simulink model "LQR_Metodo_Simulink"  (R2022a)
settings: Solver=VariableStepAuto  StartTime=0.0  StopTime=2  RelTol=1e-3
undefined symbols (not defined in the file): A, B, C, K, Ke, Kf, Kf_t
settings Model: Creator=gabri  LastModifiedBy=gabri

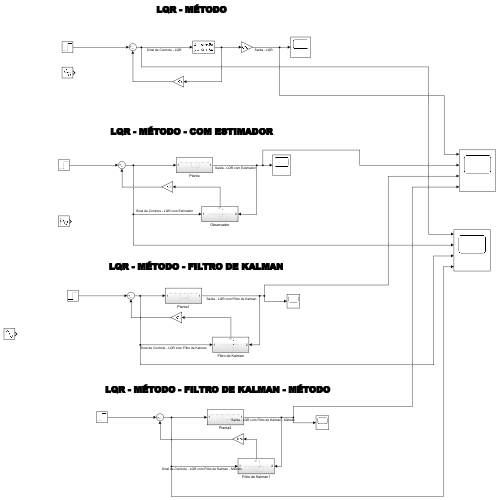
[thumbnail: Simulink's stored preview of the top-level diagram]
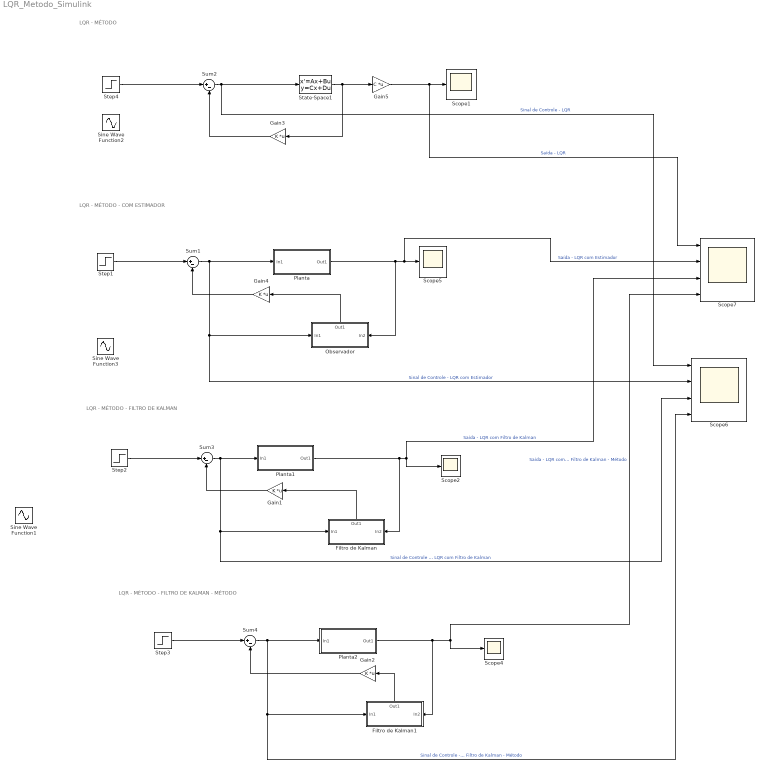
== system LQR_Metodo_Simulink ==
  note: LQR - MÉTODO
  note: LQR - MÉTODO - COM ESTIMADOR
  note: LQR - MÉTODO - FILTRO DE KALMAN
  note: LQR - MÉTODO - FILTRO DE KALMAN - MÉTODO
  Filtro de Kalman : Subsystem
      settings: PortSchema="{\"entries\":[{\"content\":{\"sides\":[{\"content\":{\"connectorIds\":[\"In1\"]},\"type\":\"ConnectorPlacement.EquallySpacedRectSide\",\"uuid\":\"a39a08db-6117-4f96-90c3-02f1f7ffb9ec\"},{\"content\":{\"connectorIds\":[\"In2\"],\"side\":\"RIGHT\"},\"type\":\"ConnectorPlacement.EquallySpacedRectSide\",\"uuid\":\"e0a0a54b-1f6f-4425-9f49-01d22204810c\"},{\"content\":{\"connectorIds\":[\"Out1\"],\"side\":\"TOP\"},\"type\":\"ConnectorPlacement.EquallySpacedRectSide\",\"uuid\":\"f9c2d93e-7541-4a9e-b077-600f0b58f20b\"},{\"content\":{\"connectorIds\":[],\"side\":\"BOTTOM\"},\"type\":\"ConnectorPlacement.EquallySpacedRectSide\",\"uuid\":\"2e0212ac-38a2-465c-9330-e4bad70b5dfc\"}]},\"type\":\"ConnectorPlacement.EquallySpacedConnector\",\"uuid\":\"106c2d4c-b59c-4d15-84b9-899fdea4a460\"}],\"packageUris\":[\"http://schema.mathworks.com/mf0/Connector/R2020b\"],\"version\":\"1.0\"}"
  Filtro de Kalman1 : Subsystem
      settings: PortSchema="{\"entries\":[{\"content\":{\"sides\":[{\"content\":{\"connectorIds\":[\"In1\"]},\"type\":\"ConnectorPlacement.EquallySpacedRectSide\",\"uuid\":\"a39a08db-6117-4f96-90c3-02f1f7ffb9ec\"},{\"content\":{\"connectorIds\":[\"In2\"],\"side\":\"RIGHT\"},\"type\":\"ConnectorPlacement.EquallySpacedRectSide\",\"uuid\":\"e0a0a54b-1f6f-4425-9f49-01d22204810c\"},{\"content\":{\"connectorIds\":[\"Out1\"],\"side\":\"TOP\"},\"type\":\"ConnectorPlacement.EquallySpacedRectSide\",\"uuid\":\"f9c2d93e-7541-4a9e-b077-600f0b58f20b\"},{\"content\":{\"connectorIds\":[],\"side\":\"BOTTOM\"},\"type\":\"ConnectorPlacement.EquallySpacedRectSide\",\"uuid\":\"2e0212ac-38a2-465c-9330-e4bad70b5dfc\"}]},\"type\":\"ConnectorPlacement.EquallySpacedConnector\",\"uuid\":\"106c2d4c-b59c-4d15-84b9-899fdea4a460\"}],\"packageUris\":[\"http://schema.mathworks.com/mf0/Connector/R2020b\"],\"version\":\"1.0\"}"
  Gain{1..4} (4 alike) : Gain  Gain=K  Multiplication=Matrix(K*u)
  Gain5 : Gain  Gain=C  Multiplication=Matrix(K*u)
  Observador : Subsystem
      settings: PortSchema="{\"entries\":[{\"content\":{\"sides\":[{\"content\":{\"connectorIds\":[\"In1\"]},\"type\":\"ConnectorPlacement.EquallySpacedRectSide\",\"uuid\":\"a39a08db-6117-4f96-90c3-02f1f7ffb9ec\"},{\"content\":{\"connectorIds\":[\"In2\"],\"side\":\"RIGHT\"},\"type\":\"ConnectorPlacement.EquallySpacedRectSide\",\"uuid\":\"e0a0a54b-1f6f-4425-9f49-01d22204810c\"},{\"content\":{\"connectorIds\":[\"Out1\"],\"side\":\"TOP\"},\"type\":\"ConnectorPlacement.EquallySpacedRectSide\",\"uuid\":\"f9c2d93e-7541-4a9e-b077-600f0b58f20b\"},{\"content\":{\"connectorIds\":[],\"side\":\"BOTTOM\"},\"type\":\"ConnectorPlacement.EquallySpacedRectSide\",\"uuid\":\"2e0212ac-38a2-465c-9330-e4bad70b5dfc\"}]},\"type\":\"ConnectorPlacement.EquallySpacedConnector\",\"uuid\":\"106c2d4c-b59c-4d15-84b9-899fdea4a460\"}],\"packageUris\":[\"http://schema.mathworks.com/mf0/Connector/R2020b\"],\"version\":\"1.0\"}"
  Planta : Subsystem
  Planta1 : Subsystem
  Planta2 : Subsystem
  Scope{1..2,4..5} (4 alike) : Scope
  Scope6 : Scope  NumInputPorts=4
  Scope7 : Scope  NumInputPorts=4
  Sine Wave Function1 : Sin  Amplitude=0.002  Frequency=pi/3  SampleTime=0
  Sine Wave Function2 : Sin  Amplitude=0.001  Frequency=pi/3  SampleTime=0
  Sine Wave Function3 : Sin  Amplitude=0.002  Frequency=pi/3  SampleTime=0
  State-Space1 : StateSpace  A=A  B=B  C=eye(3)  D=[0;0;0]  InitialCondition=0
  Step{1..4} (4 alike) : Step  Time=0  After=0.002  SampleTime=0
  Sum{1..4} (4 alike) : Sum  Inputs=|+-
  wires:
  Gain4/1 -> Sum1/2
  Observador/1(Out1) -> Gain4/1
  Sum1/1 -> Scope6/2, Observador/1(In1), Planta/1(In1)  "Sinal de Controle - LQR com Estimador"
  Gain5/1 -> Scope7/1, Scope1/1  "Saída - LQR"
  Planta/1(Out1) -> Scope7/2, Scope5/1, Observador/2(In2)  "Saída - LQR com Estimador"
  Gain3/1 -> Sum2/2
  State-Space1/1 -> Gain3/1, Gain5/1
  Sum2/1 -> Scope6/1, State-Space1/1  "Sinal de Controle - LQR"
  Filtro de Kalman/1(Out1) -> Gain1/1
  Planta1/1(Out1) -> Filtro de Kalman/2(In2), Scope7/3, Scope2/1  "Saída - LQR com Filtro de Kalman"
  Sum3/1 -> Planta1/1(In1), Scope6/3, Filtro de Kalman/1(In1)  "Sinal de Controle - LQR com Filtro de Kalman"
  Gain1/1 -> Sum3/2
  Step4/1 -> Sum2/1
  Step1/1 -> Sum1/1
  Step2/1 -> Sum3/1
  Filtro de Kalman1/1(Out1) -> Gain2/1
  Sum4/1 -> Scope6/4, Filtro de Kalman1/1(In1), Planta2/1(In1)  "Sinal de Controle - LQR com Filtro de Kalman - Método"
  Planta2/1(Out1) -> Filtro de Kalman1/2(In2), Scope7/4, Scope4/1  "Saída - LQR com Filtro de Kalman - Método"
  Gain2/1 -> Sum4/2
  Step3/1 -> Sum4/1

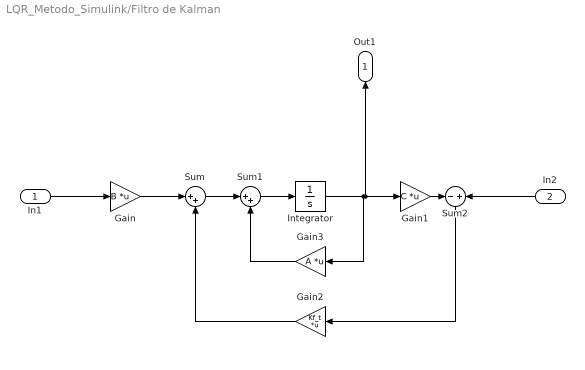
== system LQR_Metodo_Simulink/Filtro de Kalman ==
  In1 : Inport
  In2 : Inport  Port=2
  Gain : Gain  Gain=B  Multiplication=Matrix(K*u)
  Gain1 : Gain  Gain=C  Multiplication=Matrix(K*u)
  Gain2 : Gain  Gain=Kf_t  Multiplication=Matrix(K*u)
  Gain3 : Gain  Gain=A  Multiplication=Matrix(K*u)
  Integrator : Integrator
  Sum : Sum  Inputs=|++
  Sum1 : Sum  Inputs=|++
  Sum2 : Sum  Inputs=-|+
  Out1 : Outport
  wires:
  In1/1 -> Gain/1
  Gain/1 -> Sum/1
  Sum/1 -> Sum1/1
  Sum1/1 -> Integrator/1
  Integrator/1 -> Out1/1, Gain1/1, Gain3/1
  Gain1/1 -> Sum2/1
  In2/1 -> Sum2/2
  Sum2/1 -> Gain2/1
  Gain2/1 -> Sum/2
  Gain3/1 -> Sum1/2

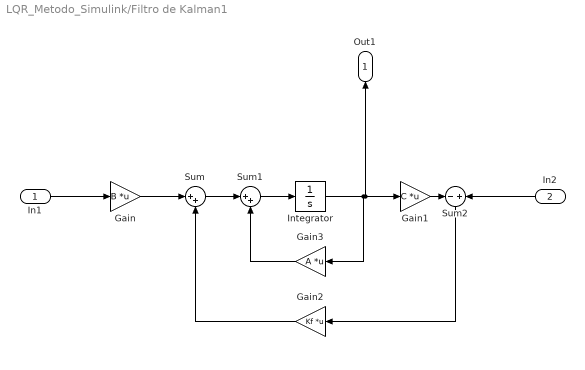
== system LQR_Metodo_Simulink/Filtro de Kalman1 ==
  In1 : Inport
  In2 : Inport  Port=2
  Gain : Gain  Gain=B  Multiplication=Matrix(K*u)
  Gain1 : Gain  Gain=C  Multiplication=Matrix(K*u)
  Gain2 : Gain  Gain=Kf  Multiplication=Matrix(K*u)
  Gain3 : Gain  Gain=A  Multiplication=Matrix(K*u)
  Integrator : Integrator
  Sum : Sum  Inputs=|++
  Sum1 : Sum  Inputs=|++
  Sum2 : Sum  Inputs=-|+
  Out1 : Outport
  wires:
  In1/1 -> Gain/1
  Gain/1 -> Sum/1
  Sum/1 -> Sum1/1
  Sum1/1 -> Integrator/1
  Integrator/1 -> Out1/1, Gain1/1, Gain3/1
  Gain1/1 -> Sum2/1
  In2/1 -> Sum2/2
  Sum2/1 -> Gain2/1
  Gain2/1 -> Sum/2
  Gain3/1 -> Sum1/2

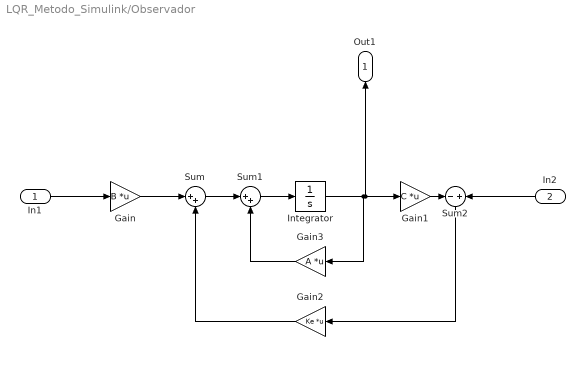
== system LQR_Metodo_Simulink/Observador ==
  In1 : Inport
  In2 : Inport  Port=2
  Gain : Gain  Gain=B  Multiplication=Matrix(K*u)
  Gain1 : Gain  Gain=C  Multiplication=Matrix(K*u)
  Gain2 : Gain  Gain=Ke  Multiplication=Matrix(K*u)
  Gain3 : Gain  Gain=A  Multiplication=Matrix(K*u)
  Integrator : Integrator
  Sum : Sum  Inputs=|++
  Sum1 : Sum  Inputs=|++
  Sum2 : Sum  Inputs=-|+
  Out1 : Outport
  wires:
  In1/1 -> Gain/1
  Gain/1 -> Sum/1
  Sum/1 -> Sum1/1
  Sum1/1 -> Integrator/1
  Integrator/1 -> Out1/1, Gain1/1, Gain3/1
  Gain1/1 -> Sum2/1
  In2/1 -> Sum2/2
  Sum2/1 -> Gain2/1
  Gain2/1 -> Sum/2
  Gain3/1 -> Sum1/2

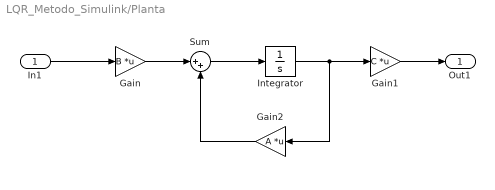
== system LQR_Metodo_Simulink/Planta ==
  In1 : Inport
  Gain : Gain  Gain=B  Multiplication=Matrix(K*u)
  Gain1 : Gain  Gain=C  Multiplication=Matrix(K*u)
  Gain2 : Gain  Gain=A  Multiplication=Matrix(K*u)
  Integrator : Integrator
  Sum : Sum  Inputs=|++
  Out1 : Outport
  wires:
  In1/1 -> Gain/1
  Gain/1 -> Sum/1
  Sum/1 -> Integrator/1
  Integrator/1 -> Gain2/1, Gain1/1
  Gain1/1 -> Out1/1
  Gain2/1 -> Sum/2

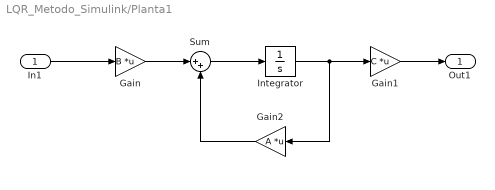
== system LQR_Metodo_Simulink/Planta1 ==
  In1 : Inport
  Gain : Gain  Gain=B  Multiplication=Matrix(K*u)
  Gain1 : Gain  Gain=C  Multiplication=Matrix(K*u)
  Gain2 : Gain  Gain=A  Multiplication=Matrix(K*u)
  Integrator : Integrator
  Sum : Sum  Inputs=|++
  Out1 : Outport
  wires:
  In1/1 -> Gain/1
  Gain/1 -> Sum/1
  Sum/1 -> Integrator/1
  Integrator/1 -> Gain2/1, Gain1/1
  Gain1/1 -> Out1/1
  Gain2/1 -> Sum/2

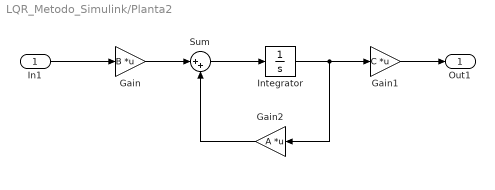
== system LQR_Metodo_Simulink/Planta2 ==
  In1 : Inport
  Gain : Gain  Gain=B  Multiplication=Matrix(K*u)
  Gain1 : Gain  Gain=C  Multiplication=Matrix(K*u)
  Gain2 : Gain  Gain=A  Multiplication=Matrix(K*u)
  Integrator : Integrator
  Sum : Sum  Inputs=|++
  Out1 : Outport
  wires:
  In1/1 -> Gain/1
  Gain/1 -> Sum/1
  Sum/1 -> Integrator/1
  Integrator/1 -> Gain2/1, Gain1/1
  Gain1/1 -> Out1/1
  Gain2/1 -> Sum/2
